simulink library "Wall_in"  (R2013b)
settings: Solver=ode45  StartTime=0.0  StopTime=10.0  RelTol=1e-3
libraries: carnot x3
settings Model: Creator=lena.frank  LastModifiedBy=drhf

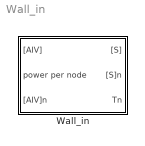
== system Wall_in ==
  Wall_in : Subsystem  mask(inner wall){wallsize=[10 10], d=[0.1 0.1 0.1], cond=[1 1 1], cwall=[0.28 0.28 0.28]*3600, rho=[2000 200 2000], emission_in=.96, dactive=[0.075 0.15 0.225], t0=10, tau=10*3600}
      mask prompts: wallsize "size of wall [m] [height width]"; d "thickness of layers [m] (vector) (0 = towards this room)"; cond "conductivity of layers [W/(m*K)] (vector)"; cwall "capacity of layers [J/(kg*K)] (vector)"; rho "density of layers [kg/m³]"; emission_in "emission of wall surface"; dactive "depth active layer in m from inner surface  (-1 = none)"; t0 "initial temperature [degree centigrade]"; tau "time-constant of wall [s]"
      mask help:
      | This is the model of an inner wall in a house.
      | first element of the vector = layer to room ([AIV], [S])
      | last element of the vector = layer to neighbour room ([AIV]n, [S]n)
      mask init:
      | position = [0 90 0 ];
      | % nodes = length(d);
      | wallheight = wallsize(1);
      | wallsurface = wallsize(1)*wallsize(2);
      | 
      | if (dactive>=0) 
      |     active = 1;
      | else
      |     active = 0;
      | end
      mask Help: web(fullfile(path_carnot('help'),'Wall_in.html'),'-helpbrowser')

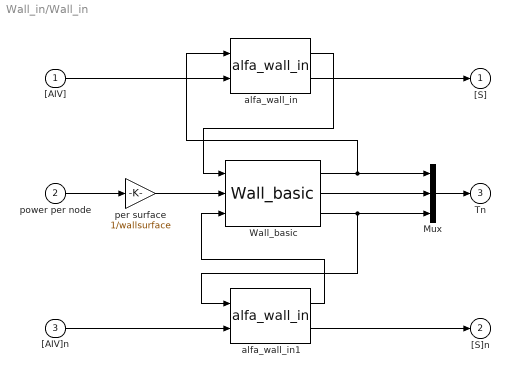
== system Wall_in/Wall_in ==
  "[AIV]" : Inport
  power per node : Inport  Port=2
  "[AIV]n" : Inport  Port=3
  Mux : Mux  Inputs=3
  Wall_basic : carnot/Basic/Thermal_Models/Wall_basic  tau=tau  t0=t0  d=d  dactive=dactive  cond=cond  cwall=cwall  rho=rho
  alfa_wall_in : carnot/Load/Houses/heat_transfer/alfa_wall_in  active=active  emission_in=emission_in  wallsurface=wallsurface
  alfa_wall_in1 : carnot/Load/Houses/heat_transfer/alfa_wall_in  active=active  emission_in=emission_in  wallsurface=wallsurface
  per surface : Gain  Gain=1/wallsurface  SaturateOnIntegerOverflow=on  OutDataTypeStr=Inherit: Same as input  ParamDataTypeStr=Inherit: Same as input
  "[S]" : Outport
  "[S]n" : Outport  Port=2
  Tn : Outport  Port=3
  wires:
  power per node/1 -> per surface/1
  per surface/1 -> Wall_basic/2
  alfa_wall_in/1 -> Wall_basic/1
  alfa_wall_in/2 -> "[S]"/1
  Wall_basic/1 -> alfa_wall_in/1, Mux/1
  "[AIV]"/1 -> alfa_wall_in/2
  alfa_wall_in1/1 -> Wall_basic/3
  Wall_basic/3 -> Mux/3, alfa_wall_in1/1
  "[AIV]n"/1 -> alfa_wall_in1/2
  alfa_wall_in1/2 -> "[S]n"/1
  Wall_basic/2 -> Mux/2
  Mux/1 -> Tn/1
